simulink model "UnicycleRobot"  (R2024b)
settings: Solver=FixedStepAuto  StartTime=0.0  StopTime=1  FixedStep=0.001  RelTol=1e-3
settings Model: Creator=elija  LastModifiedBy=elija

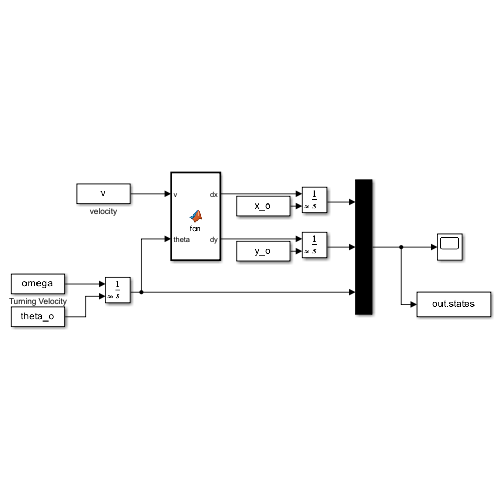
[thumbnail: Simulink's stored preview of the top-level diagram]
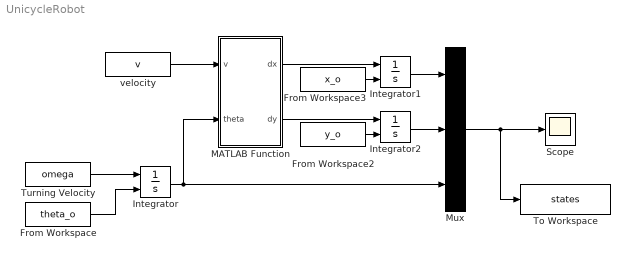
== system UnicycleRobot ==
  From Workspace : FromWorkspace  VariableName=theta_o
  From Workspace2 : FromWorkspace  VariableName=y_o
  From Workspace3 : FromWorkspace  VariableName=x_o
  Integrator : Integrator  InitialConditionSource=external
  Integrator1 : Integrator  InitialConditionSource=external
  Integrator2 : Integrator  InitialConditionSource=external
  MATLAB Function : MATLAB Function  TreatAsAtomicUnit=on
  Mux : Mux  Inputs=3
  Scope : Scope
  To Workspace : ToWorkspace  VariableName=states  SaveFormat=Timeseries  SampleTime=-1
  Turning Velocity : FromWorkspace  VariableName=omega
  velocity : FromWorkspace  VariableName=v
  wires:
  Turning Velocity/1 -> Integrator/1
  From Workspace/1 -> Integrator/2
  Integrator/1 -> Mux/3, MATLAB Function/2(theta)
  velocity/1 -> MATLAB Function/1(v)
  MATLAB Function/2(dy) -> Integrator2/1
  MATLAB Function/1(dx) -> Integrator1/1
  From Workspace2/1 -> Integrator2/2
  From Workspace3/1 -> Integrator1/2
  Integrator1/1 -> Mux/1
  Integrator2/1 -> Mux/2
  Mux/1 -> To Workspace/1, Scope/1

== matlab function UnicycleRobot/MATLAB Function ==
  data: dx output; dy output; v input; theta input
function [dx,dy] = fcn(v,theta)

dx = v.*cos(theta);
dy = v.*sin(theta);


end
